simulink model "Analog_DSSS_GC"  (R2017a)
settings: Solver=VariableStepAuto  StartTime=0.0  StopTime=50.0  RelTol=1e-3
model workspace (MAT data in the model file):
  Amp = Simulink.Parameter
  Amp.Value = [0.5 1 1.5 2]
  Amp.DataType = 'auto'
  Amp.Dimensions = [1 4]
  FreqBase = Simulink.Parameter
  FreqBase.Value = 1
  FreqBase.DataType = 'auto'
  FreqBase.Dimensions = [1 1]
  FreqCode = Simulink.Parameter
  FreqCode.Value = 0.125
  FreqCode.DataType = 'auto'
  FreqCode.Dimensions = [1 1]
  Phs = Simulink.Parameter
  Phs.Value = [0 0.785398163397 1.57079632679 2.35619449019]
  Phs.DataType = 'auto'
  Phs.Dimensions = [1 4]
values from neighbouring files (symbols this model uses):
  Amp = Simulink.Parameter    [Analog_DSSS_GC_saveas.m]    (also in Analog_DSSS_WH_saveas.m)
  FreqBase = Simulink.Parameter    [Analog_DSSS_GC_saveas.m]    (also in Analog_DSSS_WH_saveas.m)
  FreqCode = Simulink.Parameter    [Analog_DSSS_GC_saveas.m]    (also in Analog_DSSS_WH_saveas.m)
  Phs = Simulink.Parameter    [Analog_DSSS_GC_saveas.m]    (also in Analog_DSSS_WH_saveas.m)
libraries: dsparch4 x4, commseqgen3 x4, commutil2 x4
settings Model: Creator=rooki  LastModifiedBy=rooki

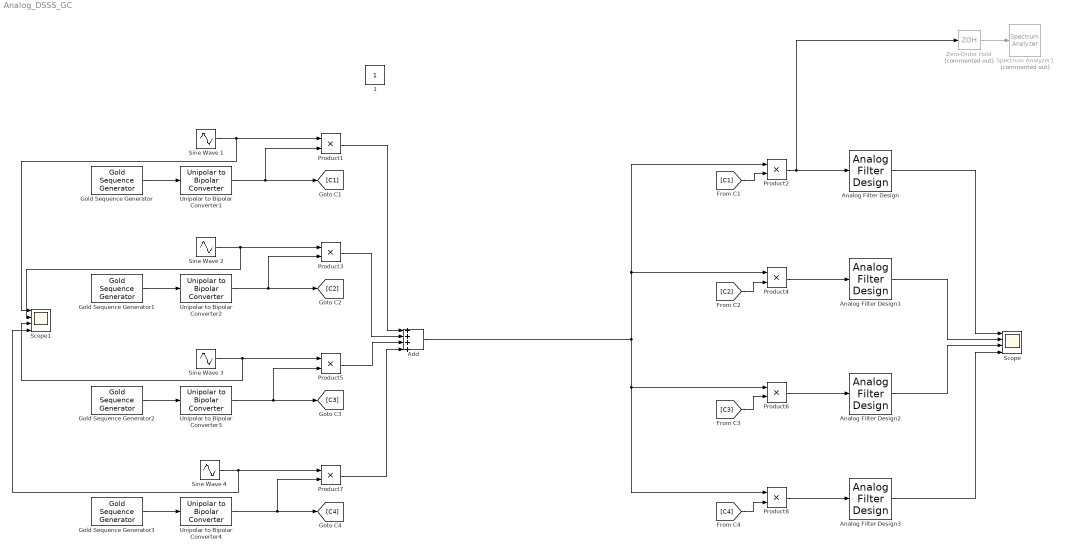
== system Analog_DSSS_GC ==
  Add : Sum  Inputs=++++
  Analog Filter Design{,1..3} (4 alike) : dsparch4/Analog Filter Design  method=Butterworth  filttype=Lowpass  N=8  Wlo=2  Whi=80  Rp=2  Rs=40
  Gold Sequence Generator : commseqgen3/Gold Sequence Generator  genPoly1='z^3 + z + 1'  iniState1=[0 0 1]  genPoly2='z^3 + z^2 + 1'  iniState2=[0 0 1]  index=0  shift=0  outVarSiz=off  maxOutSizeMode=Dialog parameter  maxOutSize=[10 1]  Ts=FreqCode  sampPerFrame=1  reset=off  outDataType=double
      settings: SourceProductName=Communications System Toolbox  SourceProductBaseCode=CM
  Gold Sequence Generator1 : commseqgen3/Gold Sequence Generator  genPoly1='z^3 + z + 1'  iniState1=[0 0 1]  genPoly2='z^3 + z^2 + 1'  iniState2=[0 1 0]  index=0  shift=0  outVarSiz=off  maxOutSizeMode=Dialog parameter  maxOutSize=[10 1]  Ts=FreqCode  sampPerFrame=1  reset=off  outDataType=double
      settings: SourceProductName=Communications System Toolbox  SourceProductBaseCode=CM
  Gold Sequence Generator2 : commseqgen3/Gold Sequence Generator  genPoly1='z^3 + z + 1'  iniState1=[0 0 1]  genPoly2='z^3 + z^2 + 1'  iniState2=[0 1 1]  index=0  shift=0  outVarSiz=off  maxOutSizeMode=Dialog parameter  maxOutSize=[10 1]  Ts=FreqCode  sampPerFrame=1  reset=off  outDataType=double
      settings: SourceProductName=Communications System Toolbox  SourceProductBaseCode=CM
  Gold Sequence Generator3 : commseqgen3/Gold Sequence Generator  genPoly1='z^3 + z + 1'  iniState1=[0 0 1]  genPoly2='z^3 + z^2 + 1'  iniState2=[1 0 0]  index=0  shift=0  outVarSiz=off  maxOutSizeMode=Dialog parameter  maxOutSize=[10 1]  Ts=FreqCode  sampPerFrame=1  reset=off  outDataType=double
      settings: SourceProductName=Communications System Toolbox  SourceProductBaseCode=CM
  Product{1..8} (8 alike) : Product
  Scope : Scope  NumInputPorts=4
  Scope1 : Scope  NumInputPorts=4
  Sine Wave 1 : Sin  Amplitude=Amp(1)  Frequency=FreqBase  Phase=Phs(1)  SampleTime=0
  Sine Wave 2 : Sin  Amplitude=Amp(2)  Frequency=FreqBase  Phase=Phs(2)  SampleTime=0
  Sine Wave 3 : Sin  Amplitude=Amp(3)  Frequency=FreqBase  Phase=Phs(3)  SampleTime=0
  Sine Wave 4 : Sin  Amplitude=Amp(4)  Frequency=FreqBase  Phase=Phs(4)  SampleTime=0
  Spectrum Analyzer1 : SpectrumAnalyzer  Commented=on
  Unipolar to Bipolar Converter{1..4} (4 alike) : commutil2/Unipolar to Bipolar Converter  M=2  polarity=Positive  dataType=Inherit via internal rule
      settings: SourceProductName=Communications System Toolbox
  Zero-Order Hold : ZeroOrderHold  Commented=on  SampleTime=-1
  1 : Constant  IOType=siggen
  wires:
  Unipolar to Bipolar Converter1/1 -> Product1/2, [C1]
  Zero-Order Hold/1 -> Spectrum Analyzer1/1
  Unipolar to Bipolar Converter2/1 -> [C2], Product3/2
  Product1/1 -> Add/1
  Product3/1 -> Add/2
  Product2/1 -> Zero-Order Hold/1, Analog Filter Design/1
  Analog Filter Design/1 -> Scope/1
  Product4/1 -> Analog Filter Design1/1
  Analog Filter Design1/1 -> Scope/2
  Product5/1 -> Add/3
  Unipolar to Bipolar Converter3/1 -> [C3], Product5/2
  Product6/1 -> Analog Filter Design2/1
  Analog Filter Design2/1 -> Scope/3
  Sine Wave 1/1 -> Scope1/1, Product1/1
  Product8/1 -> Analog Filter Design3/1
  Product7/1 -> Add/4
  Unipolar to Bipolar Converter4/1 -> [C4], Product7/2
  Analog Filter Design3/1 -> Scope/4
  Sine Wave 2/1 -> Scope1/2, Product3/1
  Sine Wave 3/1 -> Scope1/3, Product5/1
  Sine Wave 4/1 -> Scope1/4, Product7/1
  [C1] -> Product2/2
  [C2] -> Product4/2
  [C3] -> Product6/2
  [C4] -> Product8/2
  Gold Sequence Generator/1 -> Unipolar to Bipolar Converter1/1
  Gold Sequence Generator1/1 -> Unipolar to Bipolar Converter2/1
  Gold Sequence Generator2/1 -> Unipolar to Bipolar Converter3/1
  Gold Sequence Generator3/1 -> Unipolar to Bipolar Converter4/1
  Add/1 -> Product8/1, Product6/1, Product4/1, Product2/1
